simulink model "Overall_Mission"  (R2023a)
settings: Solver=VariableStepAuto  StartTime=0.0  StopTime=10.0  RelTol=1e-3
PreLoadFcn:
  | load AllBuses
settings Model: Creator=rose  LastModifiedBy=rose
settings OptimizationCC: DefaultParameterBehavior=Inlined

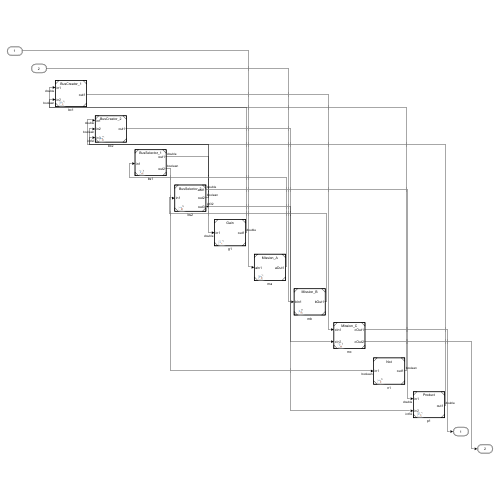
[thumbnail: Simulink's stored preview of the top-level diagram]
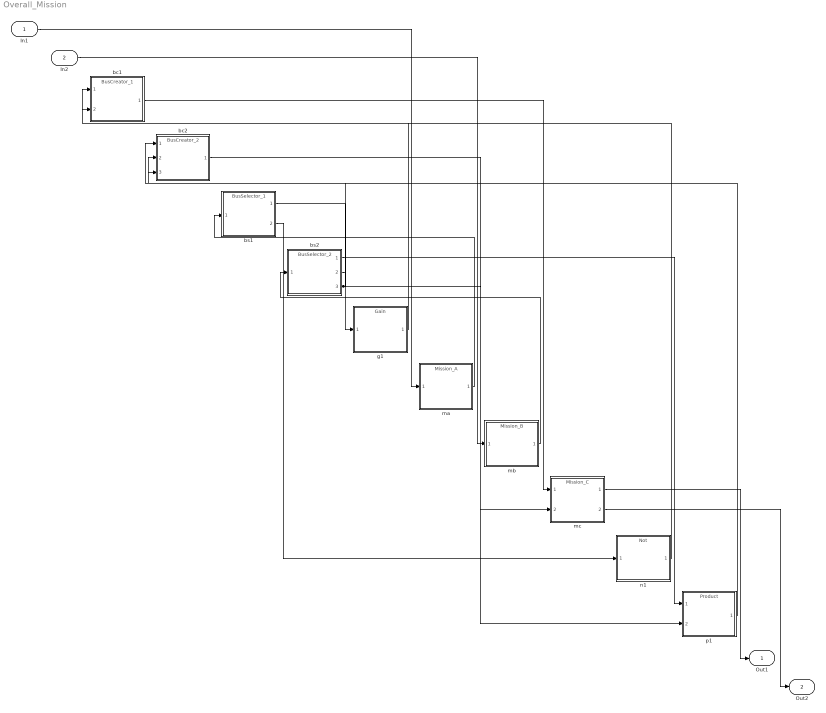
== system Overall_Mission ==
  In1 : Inport  OutDataTypeStr=Bus: Bus_1  BusOutputAsStruct=on
  In2 : Inport  Port=2  OutDataTypeStr=Bus: Bus_2  BusOutputAsStruct=on
  bc1 : ModelReference  ModelNameDialog=BusCreator_1  SimulationMode=Normal  ModelReferenceVersion=1.1
  bc2 : ModelReference  ModelNameDialog=BusCreator_2  SimulationMode=Normal  ModelReferenceVersion=1.1
  bs1 : ModelReference  ModelNameDialog=BusSelector_1  SimulationMode=Normal  ModelReferenceVersion=1.1
  bs2 : ModelReference  ModelNameDialog=BusSelector_2  SimulationMode=Normal  ModelReferenceVersion=1.1
  g1 : ModelReference  ModelNameDialog=Gain  SimulationMode=Normal  ModelReferenceVersion=1.1
  ma : ModelReference  ModelNameDialog=Mission_A  SimulationMode=Normal  ModelReferenceVersion=1.1
  mb : ModelReference  ModelNameDialog=Mission_B  SimulationMode=Normal  ModelReferenceVersion=1.1
  mc : ModelReference  ModelNameDialog=Mission_C  SimulationMode=Normal  ModelReferenceVersion=1.1
  n1 : ModelReference  ModelNameDialog=Not  SimulationMode=Normal  ModelReferenceVersion=1.1
  p1 : ModelReference  ModelNameDialog=Product  SimulationMode=Normal  ModelReferenceVersion=1.1
  Out1 : Outport  OutDataTypeStr=Bus: Bus_1  BusOutputAsStruct=on
  Out2 : Outport  Port=2  OutDataTypeStr=Bus: Bus_1  BusOutputAsStruct=on
  wires:
  bc1/1 -> mc/1
  bc2/1 -> mc/2
  bs1/1 -> g1/1
  bs1/2 -> n1/1
  bs2/1 -> p1/1
  bs2/2 -> bc2/2
  bs2/3 -> bc2/3, p1/2
  g1/1 -> bc1/1
  In1/1 -> ma/1
  In2/1 -> mb/1
  ma/1 -> bs1/1
  mb/1 -> bs2/1
  mc/1 -> Out1/1
  mc/2 -> Out2/1
  n1/1 -> bc1/2
  p1/1 -> bc2/1
